simulink model "oya2"  (R2015b)
settings: Solver=ode45  StartTime=0.0  StopTime=20  RelTol=1e-3
settings Model: Creator=yusuke  LastModifiedBy=yuji
settings DataIOCC: SaveFormat=Array
settings HardwareCC: ProdBitPerPointer=32  ProdLargestAtomicFloat=None  ProdIntDivRoundTo=Undefined  ProdEndianess=Unspecified  ProdWordSize=32  ProdHWDeviceType=32-bit Generic
settings GRTTargetCC: GeneratePreprocessorConditionals=Disable all
settings ConfigComp: CovModelRefEnable=Off

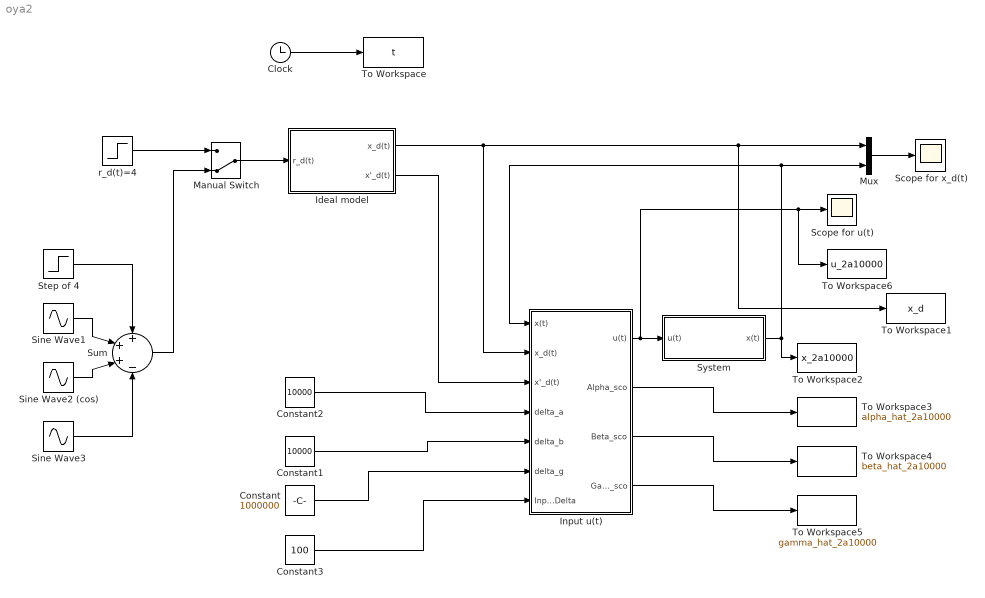
== system oya2 ==
  Clock : Clock
  Constant : Constant  Value=1000000
  Constant1 : Constant  Value=10000
  Constant2 : Constant  Value=10000
  Constant3 : Constant  Value=100
  Ideal model : Subsystem
  Input u(t) : Subsystem
  Manual Switch : ManualSwitch  CurrentSetting=0
  Mux : Mux  Inputs=2
  Scope for u(t) : Scope
  Scope for x_d(t) : Scope
  Sine Wave1 : Sin  Amplitude=0.5  Frequency=0.5  SampleTime=0.01
  Sine Wave2 (cos) : Sin  Frequency=3  Phase=pi/2  SampleTime=0.01
  Sine Wave3 : Sin  Amplitude=2  Frequency=5  SampleTime=0.01
  Step of 4 : Step  Time=0  After=4  SampleTime=0.01
  Sum : Sum  Inputs=+++-
  System : Subsystem
  To Workspace : ToWorkspace  VariableName=t  SampleTime=-1
  To Workspace1 : ToWorkspace  VariableName=x_d  SaveFormat=Timeseries  SampleTime=-1
  To Workspace2 : ToWorkspace  VariableName=x_2a10000  SaveFormat=Timeseries  SampleTime=-1
  To Workspace3 : ToWorkspace  VariableName=alpha_hat_2a10000  SaveFormat=Timeseries  SampleTime=-1
  To Workspace4 : ToWorkspace  VariableName=beta_hat_2a10000  SaveFormat=Timeseries  SampleTime=-1
  To Workspace5 : ToWorkspace  VariableName=gamma_hat_2a10000  SaveFormat=Timeseries  SampleTime=-1
  To Workspace6 : ToWorkspace  VariableName=u_2a10000  SaveFormat=Timeseries  SampleTime=-1
  r_d(t)=4 : Step  Time=0  After=4  SampleTime=0.01
  wires:
  Manual Switch/1 -> Ideal model/1(r_d(t))
  Clock/1 -> To Workspace/1
  Mux/1 -> Scope for x_d(t)/1
  Ideal model/1(x_d(t)) -> Input u(t)/2(x_d(t)), To Workspace1/1, Mux/1
  System/1(x(t)) -> Input u(t)/1(x(t)), Mux/2, To Workspace2/1
  Input u(t)/1(u(t)) -> To Workspace6/1, Scope for u(t)/1, System/1(u(t))
  Input u(t)/2(Alpha_sco) -> To Workspace3/1
  Input u(t)/3(Beta_sco) -> To Workspace4/1
  Input u(t)/4(Gamma_sco) -> To Workspace5/1
  Ideal model/2(x'_d(t)) -> Input u(t)/3(x'_d(t))
  Constant3/1 -> Input u(t)/7(Input_Delta)
  Constant/1 -> Input u(t)/6(delta_g)
  Constant1/1 -> Input u(t)/5(delta_b)
  Constant2/1 -> Input u(t)/4(delta_a)
  r_d(t)=4/1 -> Manual Switch/1
  Sum/1 -> Manual Switch/2
  Step of 4/1 -> Sum/1
  Sine Wave1/1 -> Sum/2
  Sine Wave2 (cos)/1 -> Sum/3
  Sine Wave3/1 -> Sum/4

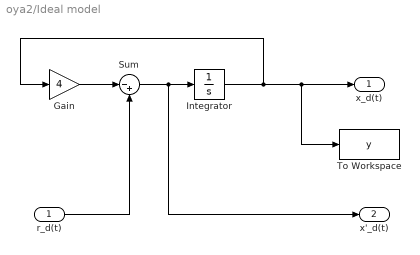
== system oya2/Ideal model ==
  r_d(t) : Inport
  Gain : Gain  Gain=4
  Integrator : Integrator
  Sum : Sum  Inputs=|-+
  To Workspace : ToWorkspace  VariableName=y  SaveFormat=Timeseries  SampleTime=-1
  x_d(t) : Outport
  x'_d(t) : Outport  Port=2
  wires:
  Integrator/1 -> Gain/1, To Workspace/1, x_d(t)/1
  Sum/1 -> x'_d(t)/1, Integrator/1
  r_d(t)/1 -> Sum/2
  Gain/1 -> Sum/1

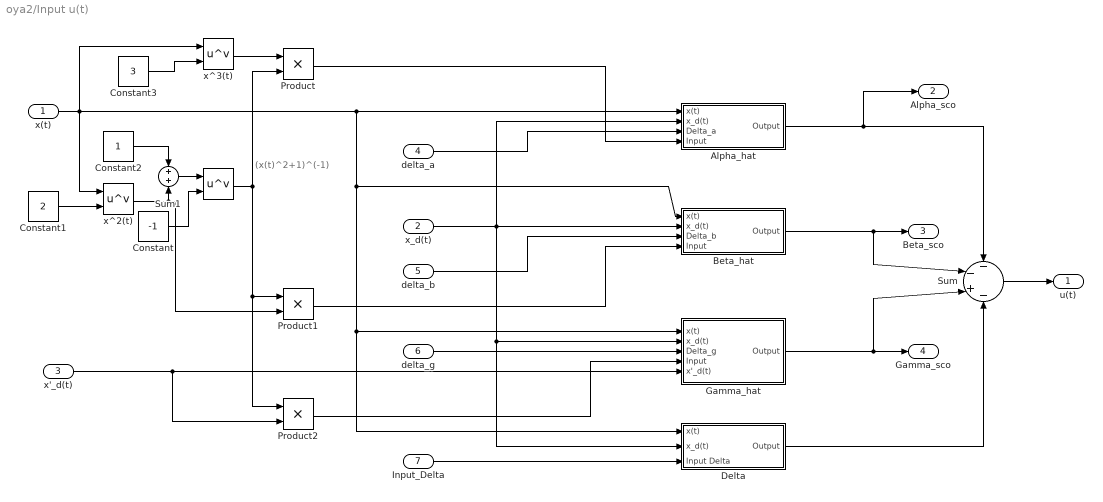
== system oya2/Input u(t) ==
  note: (x(t)^2+1)^(-1)
  x(t) : Inport
  x_d(t) : Inport  Port=2
  x'_d(t) : Inport  Port=3
  delta_a : Inport  Port=4
  delta_b : Inport  Port=5
  delta_g : Inport  Port=6
  Input_Delta : Inport  Port=7
  " " : Math  Operator=pow  SaturateOnIntegerOverflow=on
  " x^2(t)" : Math  Operator=pow  SaturateOnIntegerOverflow=on
  " x^3(t)" : Math  Operator=pow  SaturateOnIntegerOverflow=on
  Alpha_hat : Subsystem
  Beta_hat : Subsystem
  Constant : Constant  Value=-1
  Constant1 : Constant  Value=2
  Constant2 : Constant
  Constant3 : Constant  Value=3
  Delta : Subsystem
  Gamma_hat : Subsystem
  Product : Product
  Product1 : Product
  Product2 : Product
  Sum : Sum  Inputs=--+-
  Sum1 : Sum  Inputs=+|+
  u(t) : Outport
  Alpha_sco : Outport  Port=2
  Beta_sco : Outport  Port=3
  Gamma_sco : Outport  Port=4
  wires:
  Sum/1 -> u(t)/1
  Delta/1("Output ") -> Sum/4
  Gamma_hat/1(Output) -> Gamma_sco/1, Sum/3
  Beta_hat/1(Output) -> Beta_sco/1, Sum/2
  Alpha_hat/1(Output) -> Alpha_sco/1, Sum/1
  x(t)/1 -> Alpha_hat/1(x(t)), Delta/1(x(t)), Gamma_hat/1(x(t)), Beta_hat/1(x(t)), " x^3(t)"/1, " x^2(t)"/1
  x_d(t)/1 -> Gamma_hat/2(x_d(t)), Delta/2(x_d(t)), Beta_hat/2(x_d(t)), Alpha_hat/2(x_d(t))
  delta_a/1 -> Alpha_hat/3(Delta_a)
  delta_b/1 -> Beta_hat/3(Delta_b)
  delta_g/1 -> Gamma_hat/3(Delta_g)
  x'_d(t)/1 -> Product2/2, Gamma_hat/5(x'_d(t))
  Input_Delta/1 -> Delta/3(Input Delta)
  Constant/1 -> " "/2
  Constant1/1 -> " x^2(t)"/2
  Constant2/1 -> Sum1/1
  Sum1/1 -> " "/1
  Constant3/1 -> " x^3(t)"/2
  " x^3(t)"/1 -> Product/1
  " "/1 -> Product/2, Product2/1, Product1/1
  Product/1 -> Alpha_hat/4(Input)
  Product1/1 -> Beta_hat/4(Input)
  Product2/1 -> Gamma_hat/4(Input)
  " x^2(t)"/1 -> Product1/2, Sum1/2

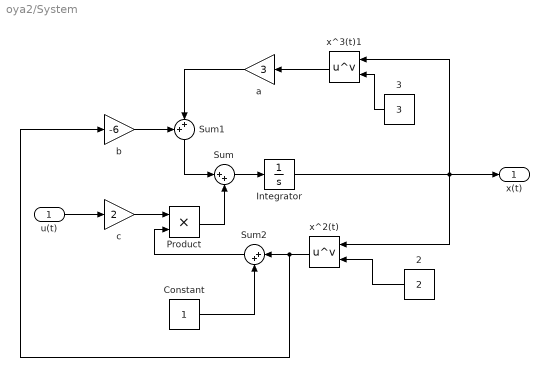
== system oya2/System ==
  u(t) : Inport
  2 : Constant  Value=2
  3 : Constant  Value=3
  Constant : Constant
  Integrator : Integrator
  Product : Product
  Sum : Sum  Inputs=|++
  Sum1 : Sum  Inputs=++|
  Sum2 : Sum  Inputs=|++
  a : Gain  Gain=3
  b : Gain  Gain=-6
  c : Gain  Gain=2
  x^2(t) : Math  Operator=pow  SaturateOnIntegerOverflow=on
  x^3(t)1 : Math  Operator=pow  SaturateOnIntegerOverflow=on
  x(t) : Outport
  wires:
  u(t)/1 -> c/1
  Integrator/1 -> x^2(t)/1, x^3(t)1/1, x(t)/1
  2/1 -> x^2(t)/2
  3/1 -> x^3(t)1/2
  Sum/1 -> Integrator/1
  Product/1 -> Sum/2
  c/1 -> Product/1
  Sum1/1 -> Sum/1
  b/1 -> Sum1/1
  x^2(t)/1 -> b/1, Sum2/1
  Sum2/1 -> Product/2
  x^3(t)1/1 -> a/1
  a/1 -> Sum1/2
  Constant/1 -> Sum2/2

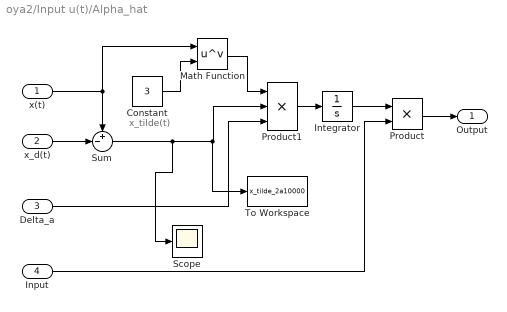
== system oya2/Input u(t)/Alpha_hat ==
  note: x_tilde(t)
  x(t) : Inport
  x_d(t) : Inport  Port=2
  Delta_a : Inport  Port=3
  Input : Inport  Port=4
  Constant : Constant  Value=3
  Integrator : Integrator
  Math Function : Math  Operator=pow  SaturateOnIntegerOverflow=on
  Product : Product
  Product1 : Product  Inputs=3
  Scope : Scope
  Sum : Sum  Inputs=+-|
  To Workspace : ToWorkspace  VariableName=x_tilde_2a10000  SaveFormat=Timeseries  SampleTime=-1
  Output : Outport
  wires:
  Product/1 -> Output/1
  Input/1 -> Product/2
  Integrator/1 -> Product/1
  Product1/1 -> Integrator/1
  Delta_a/1 -> Product1/3
  x_d(t)/1 -> Sum/2
  Sum/1 -> To Workspace/1, Product1/2, Scope/1
  x(t)/1 -> Sum/1, Math Function/1
  Constant/1 -> Math Function/2
  Math Function/1 -> Product1/1

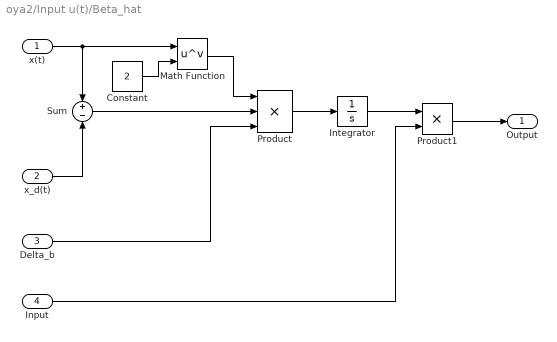
== system oya2/Input u(t)/Beta_hat ==
  x(t) : Inport
  x_d(t) : Inport  Port=2
  Delta_b : Inport  Port=3
  Input : Inport  Port=4
  Constant : Constant  Value=2
  Integrator : Integrator
  Math Function : Math  Operator=pow  SaturateOnIntegerOverflow=on
  Product : Product  Inputs=3
  Product1 : Product
  Sum : Sum  Inputs=+|-
  Output : Outport
  wires:
  x(t)/1 -> Math Function/1, Sum/1
  x_d(t)/1 -> Sum/2
  Sum/1 -> Product/2
  Delta_b/1 -> Product/3
  Product/1 -> Integrator/1
  Integrator/1 -> Product1/1
  Product1/1 -> Output/1
  Input/1 -> Product1/2
  Constant/1 -> Math Function/2
  Math Function/1 -> Product/1

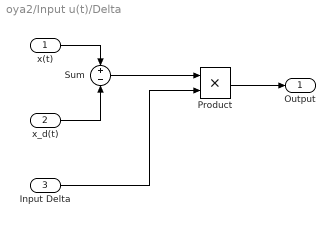
== system oya2/Input u(t)/Delta ==
  x(t) : Inport
  x_d(t) : Inport  Port=2
  Input Delta : Inport  Port=3
  Product : Product
  Sum : Sum  Inputs=+|-
  "Output " : Outport
  wires:
  x(t)/1 -> Sum/1
  x_d(t)/1 -> Sum/2
  Sum/1 -> Product/1
  Product/1 -> "Output "/1
  Input Delta/1 -> Product/2

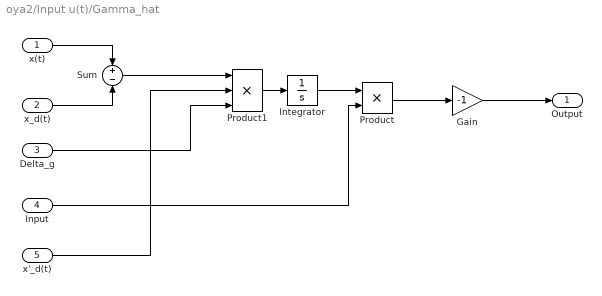
== system oya2/Input u(t)/Gamma_hat ==
  x(t) : Inport
  x_d(t) : Inport  Port=2
  Delta_g : Inport  Port=3
  Input : Inport  Port=4
  x'_d(t) : Inport  Port=5
  Gain : Gain  Gain=-1
  Integrator : Integrator
  Product : Product
  Product1 : Product  Inputs=3
  Sum : Sum  Inputs=+|-
  Output : Outport
  wires:
  x(t)/1 -> Sum/1
  x_d(t)/1 -> Sum/2
  Integrator/1 -> Product/1
  Input/1 -> Product/2
  Product1/1 -> Integrator/1
  Sum/1 -> Product1/1
  Delta_g/1 -> Product1/3
  Product/1 -> Gain/1
  Gain/1 -> Output/1
  x'_d(t)/1 -> Product1/2
